simulink model "zad3_inne_param"  (R2016b)
settings: Solver=VariableStepAuto  StartTime=0.0  StopTime=100  RelTol=1e-3
undefined symbols (not defined in the file or in its folder): Tp
settings Model: Creator=tomasz  LastModifiedBy=tomasz

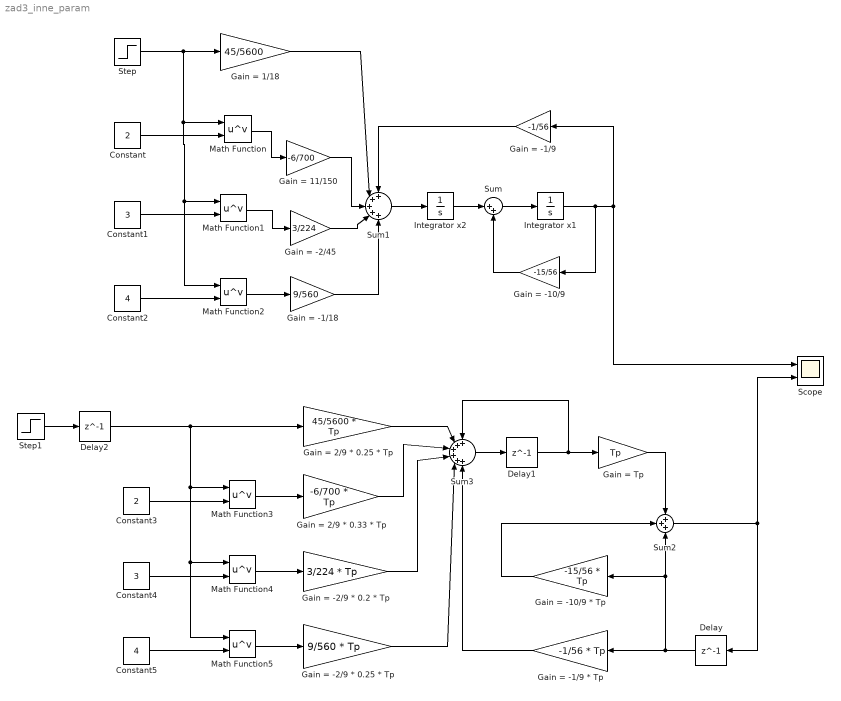
== system zad3_inne_param ==
  Constant : Constant  Value=2
  Constant1 : Constant  Value=3
  Constant2 : Constant  Value=4
  Constant3 : Constant  Value=2
  Constant4 : Constant  Value=3
  Constant5 : Constant  Value=4
  Delay : Delay  DelayLength=1  InitialCondition=0  SampleTime=Tp
  Delay1 : Delay  DelayLength=1  InitialCondition=0  SampleTime=Tp
  Delay2 : Delay  DelayLength=1  InitialCondition=0  SampleTime=Tp
  Gain = -1/18 : Gain  Gain=9/560
  Gain = -1/9 : Gain  Gain=-1/56
  Gain = -1/9 * Tp : Gain  Gain=-1/56 * Tp
  Gain = -10/9 : Gain  Gain=-15/56
  Gain = -10/9 * Tp : Gain  Gain=-15/56 * Tp
  Gain = -2/45 : Gain  Gain=3/224
  Gain = -2/9 * 0.2 * Tp : Gain  Gain=3/224 * Tp
  Gain = -2/9 * 0.25 * Tp : Gain  Gain=9/560 * Tp
  Gain = 1/18 : Gain  Gain=45/5600
  Gain = 11/150 : Gain  Gain=-6/700
  Gain = 2/9 * 0.25 * Tp : Gain  Gain=45/5600 * Tp
  Gain = 2/9 * 0.33 * Tp : Gain  Gain=-6/700 * Tp
  Gain = Tp : Gain  Gain=Tp
  Integrator x1 : Integrator
  Integrator x2 : Integrator
  Math Function{,1..5} (6 alike) : Math  Operator=pow  SaturateOnIntegerOverflow=on
  Scope : Scope  NumInputPorts=2
  Step : Step  SampleTime=0
  Step1 : Step  SampleTime=Tp
  Sum : Sum  Inputs=|++
  Sum1 : Sum  Inputs=+++++
  Sum2 : Sum  Inputs=+++
  Sum3 : Sum  Inputs=++++++
  wires:
  Sum/1 -> Integrator x1/1
  Integrator x1/1 -> Scope/1, Gain = -1/9/1, Gain = -10/9/1
  Gain = -10/9/1 -> Sum/2
  Integrator x2/1 -> Sum/1
  Sum1/1 -> Integrator x2/1
  Gain = -1/9/1 -> Sum1/1
  Step/1 -> Math Function/1, Math Function2/1, Math Function1/1, Gain = 1/18/1
  Gain = 1/18/1 -> Sum1/2
  Constant1/1 -> Math Function1/2
  Constant2/1 -> Math Function2/2
  Constant/1 -> Math Function/2
  Math Function2/1 -> Gain = -1/18/1
  Math Function1/1 -> Gain = -2/45/1
  Math Function/1 -> Gain = 11/150/1
  Gain = 11/150/1 -> Sum1/3
  Gain = -2/45/1 -> Sum1/4
  Gain = -1/18/1 -> Sum1/5
  Delay/1 -> Sum2/3, Gain = -10/9 * Tp/1, Gain = -1/9 * Tp/1
  Sum2/1 -> Scope/2, Delay/1
  Gain = -10/9 * Tp/1 -> Sum2/2
  Sum3/1 -> Delay1/1
  Delay1/1 -> Sum3/1, Gain = Tp/1
  Gain = Tp/1 -> Sum2/1
  Gain = -1/9 * Tp/1 -> Sum3/6
  Constant5/1 -> Math Function5/2
  Constant4/1 -> Math Function4/2
  Constant3/1 -> Math Function3/2
  Delay2/1 -> Math Function5/1, Math Function4/1, Math Function3/1, Gain = 2/9 * 0.25 * Tp/1
  Gain = 2/9 * 0.25 * Tp/1 -> Sum3/2
  Math Function3/1 -> Gain = 2/9 * 0.33 * Tp/1
  Gain = 2/9 * 0.33 * Tp/1 -> Sum3/3
  Math Function5/1 -> Gain = -2/9 * 0.25 * Tp/1
  Math Function4/1 -> Gain = -2/9 * 0.2 * Tp/1
  Gain = -2/9 * 0.2 * Tp/1 -> Sum3/4
  Gain = -2/9 * 0.25 * Tp/1 -> Sum3/5
  Step1/1 -> Delay2/1
